simulink model "compareModels"  (R2019a)
settings: Solver=ode45  StartTime=0.0  StopTime=SimulationTime  FixedStep=0.0001  MaxStep=maxstep  RelTol=reltol
settings Model: Creator=000  LastModifiedBy=000
settings SolverCC: MaxConsecutiveMinStep=100
settings OptimizationCC: EfficientMapNaN2IntZero=off
settings HardwareCC: TargetBitPerPointer=64  TargetBitPerSizeT=64  TargetBitPerPtrDiffT=64  TargetLongLongMode=on  TargetIntDivRoundTo=Zero  TargetEndianess=LittleEndian  TargetWordSize=64  TargetHWDeviceType=MATLAB Host  ProdEqTarget=off
settings CodeAppCC: MaxIdLength=128
settings GRTTargetCC: TargetLangStandard=C89/C90 (ANSI)  GRTInterface=on

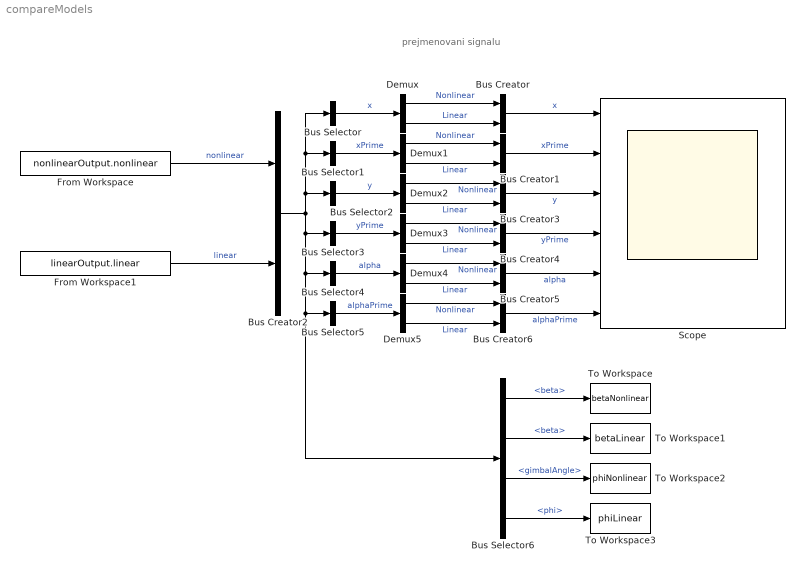
== system compareModels ==
  note: prejmenovani signalu
  Bus Creator{,1..6} (7 alike) : BusCreator  Inputs=2
  Bus Selector : BusSelector  OutputSignals=nonlinear.x,linear.x  OutputAsBus=on
  Bus Selector1 : BusSelector  OutputSignals=nonlinear.xPrime,linear.xPrime  OutputAsBus=on
  Bus Selector2 : BusSelector  OutputSignals=nonlinear.y,linear.y  OutputAsBus=on
  Bus Selector3 : BusSelector  OutputSignals=nonlinear.yPrime,linear.yPrime  OutputAsBus=on
  Bus Selector4 : BusSelector  OutputSignals=nonlinear.alpha,linear.alpha  OutputAsBus=on
  Bus Selector5 : BusSelector  OutputSignals=nonlinear.alphaPrime,linear.alphaPrime  OutputAsBus=on
  Bus Selector6 : BusSelector  OutputSignals=nonlinear.beta,linear.beta,nonlinear.gimbalAngle,linear.phi
  Demux{,1..5} (6 alike) : Demux  Outputs=2
  From Workspace : FromWorkspace  VariableName=nonlinearOutput.nonlinear  OutDataTypeStr=Bus: slBus1  SampleTime=0
  From Workspace1 : FromWorkspace  VariableName=linearOutput.linear  OutDataTypeStr=Bus: slBus2  SampleTime=0
  Scope : Scope  NumInputPorts=6
  To Workspace : ToWorkspace  VariableName=betaNonlinear  SaveFormat=Timeseries  SampleTime=-1
  To Workspace1 : ToWorkspace  VariableName=betaLinear  SaveFormat=Timeseries  SampleTime=-1
  To Workspace2 : ToWorkspace  VariableName=phiNonlinear  SaveFormat=Timeseries  SampleTime=-1
  To Workspace3 : ToWorkspace  VariableName=phiLinear  SaveFormat=Timeseries  SampleTime=-1
  wires:
  Bus Creator2/1 -> Bus Selector6/1, Bus Selector5/1, Bus Selector4/1, Bus Selector3/1, Bus Selector1/1, Bus Selector/1, Bus Selector2/1
  From Workspace/1 -> Bus Creator2/1  "nonlinear"
  From Workspace1/1 -> Bus Creator2/2  "linear"
  Bus Selector6/1 -> To Workspace/1  "<beta>"
  Bus Selector6/2 -> To Workspace1/1  "<beta>"
  Bus Selector6/4 -> To Workspace3/1  "<phi>"
  Bus Selector6/3 -> To Workspace2/1  "<gimbalAngle>"
  Bus Creator/1 -> Scope/1  "x"
  Bus Selector/1 -> Demux/1  "x"
  Demux/2 -> Bus Creator/2  "Linear"
  Demux/1 -> Bus Creator/1  "Nonlinear"
  Bus Creator1/1 -> Scope/2  "xPrime"
  Demux1/1 -> Bus Creator1/1  "Nonlinear"
  Demux1/2 -> Bus Creator1/2  "Linear"
  Bus Selector1/1 -> Demux1/1  "xPrime"
  Bus Creator3/1 -> Scope/3  "y"
  Demux2/1 -> Bus Creator3/1  "Nonlinear"
  Demux2/2 -> Bus Creator3/2  "Linear"
  Bus Selector2/1 -> Demux2/1  "y"
  Bus Creator4/1 -> Scope/4  "yPrime"
  Demux3/1 -> Bus Creator4/1  "Nonlinear"
  Demux3/2 -> Bus Creator4/2  "Linear"
  Bus Selector3/1 -> Demux3/1  "yPrime"
  Bus Creator5/1 -> Scope/5  "alpha"
  Demux4/1 -> Bus Creator5/1  "Nonlinear"
  Demux4/2 -> Bus Creator5/2  "Linear"
  Bus Selector4/1 -> Demux4/1  "alpha"
  Bus Creator6/1 -> Scope/6  "alphaPrime"
  Demux5/1 -> Bus Creator6/1  "Nonlinear"
  Demux5/2 -> Bus Creator6/2  "Linear"
  Bus Selector5/1 -> Demux5/1  "alphaPrime"
